simulink model "stage1"  (Simulink 7.7)
settings: Solver=ode45  StartTime=0.0  StopTime=20  RelTol=1e-3
libraries: powerlib x3
settings Model: Creator=Vikas  LastModifiedBy=HASANTH

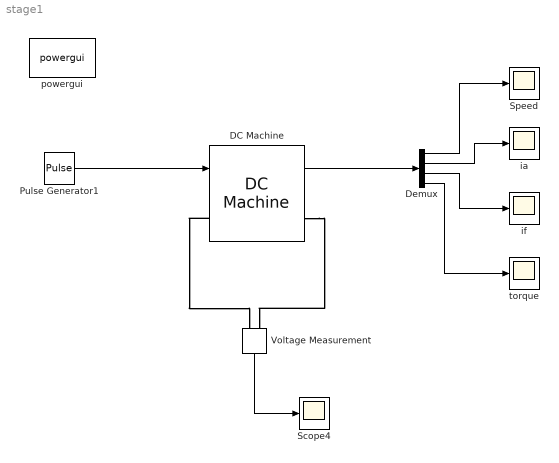
== system stage1 ==
  DC Machine : powerlib/Machines/DC Machine  SystemSampleTime=-1  PresetModel=No  MechanicalLoad=Speed w  FieldType=Permanent magnet  ShowDetailedParameters=on  RLa="[ 1  0.012]"  RLf="[ 240  120]"  Laf=1.8  MachineConstant=Back-emf constant (V/rpm)  Ke=3  Kt=3.18  J=1  Bm=0  Tf=0  w0=1  Ifinit=1  TsPowergui=0  TsBlock=-1
      settings: AttributesFormatString=\n
  Demux : Demux
  Pulse Generator1 : DiscretePulseGenerator  PulseType=Time based  Amplitude=5.4  Period=10  PulseWidth=50
  Scope4 : Scope
      settings: TimeRange=1  YMin=-15  YMax=30  SaveName=ScopeData4
  Speed : Scope
  Voltage Measurement : powerlib/Measurements/Voltage Measurement  SystemSampleTime=-1  PhasorSimulation=off  OutputType=Complex  PSBequivalent=0
  ia : Scope
  if : Scope
      settings: SaveName=ScopeData2
  powergui : powerlib/powergui  Priority=1  SystemSampleTime=-1  SimulationMode=Continuous  SampleTime=50e-6  frequency=60  SPID=off  DisableSnubberDevices=off  DisableRonSwitches=off  DisableVfSwitches=off  SwTol=0  Interpol=off  DisplayEquations=off  FunctionMessages=off  frequencyindice=0  Pbase=100e6  ErrMax=1e-4  Iterations=50  UnitsV=kV  UnitsW=MW  echomessages=off  HookPort=off  EnableUseOfTLC=off  x0status=blocks  RestoreLinks=warning  ResistiveCurrentMeasurement=off  Ylog=off  Xlog=on  ShowGrid=off  save=off  variable=ZData  ZoomFFT=off  StartTime=0.0  cycles=1  DisplayStyle=1  FreqAxis=off  MaxFrequency=1000  frequencyindicesteady=1  display=off  methode=off
  torque : Scope
      settings: SaveName=ScopeData3
  wires:
  DC Machine/1 -> Demux/1
  Demux/1 -> Speed/1
  Demux/2 -> ia/1
  Demux/3 -> if/1
  Demux/4 -> torque/1
  Voltage Measurement/1 -> Scope4/1
  Pulse Generator1/1 -> DC Machine/1
  connections:
  DC Machine/LConn1 -- Voltage Measurement/LConn1
  DC Machine/RConn1 -- Voltage Measurement/LConn2
